simulink model "model06b"  (R2018b)
settings: Solver=ode4  StartTime=0.0  StopTime=30  FixedStep=0.0001  RelTol=1e-3
values from neighbouring files (symbols this model uses):
  A_sys = [0    1 ... (first row only)    [main.m]
  B_sys = [b1 ... (first row only)    [main.m]
  C_sys = [1 0]    [main.m]
  D_sys = 0    [main.m]
  init_conds = [  0,   0 ... (first row only)    [data.m]
  k1 = b^2/((V^2*sin(lambda)-b*g*cos(lambda))*m*a*c*sin(lambda))    [main.m]
  k2 = b*g/(V^2*sin(lambda)-b*g*cos(lambda))    [main.m]
undefined symbols (not defined in the file or in its folder): denK, numK
settings Model: Creator=franc  LastModifiedBy=franc

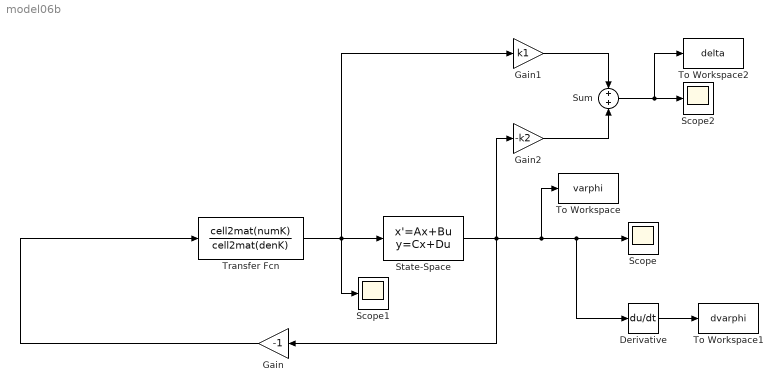
== system model06b ==
  Derivative : Derivative
  Gain : Gain  Gain=-1
  Gain1 : Gain  Gain=k1
  Gain2 : Gain  Gain=-k2
  Scope : Scope
  Scope1 : Scope
  Scope2 : Scope
  State-Space : StateSpace  A=A_sys  B=B_sys  C=C_sys  D=D_sys  InitialCondition=init_conds(2, :)
  Sum : Sum  Inputs=+|+
  To Workspace : ToWorkspace  VariableName=varphi  SaveFormat=Timeseries  SampleTime=-1
  To Workspace1 : ToWorkspace  VariableName=dvarphi  SaveFormat=Timeseries  SampleTime=-1
  To Workspace2 : ToWorkspace  VariableName=delta  SaveFormat=Timeseries  SampleTime=-1
  Transfer Fcn : TransferFcn  Numerator=cell2mat(numK)  Denominator=cell2mat(denK)
  wires:
  Transfer Fcn/1 -> Scope1/1, Gain1/1, State-Space/1
  State-Space/1 -> Gain/1, To Workspace/1, Derivative/1, Scope/1, Gain2/1
  Gain/1 -> Transfer Fcn/1
  Gain1/1 -> Sum/1
  Gain2/1 -> Sum/2
  Sum/1 -> To Workspace2/1, Scope2/1
  Derivative/1 -> To Workspace1/1
